simulink model "ModelConveyorWithLogic"  (R2020b)
settings: Solver=FixedStepAuto  StartTime=0.0  StopTime=Inf  FixedStep=0.010  RelTol=1e-3
libraries: simulink x2
settings Model: Creator=kaebi  LastModifiedBy=kaebi
settings OptimizationCC: DefaultParameterBehavior=Inlined  LocalBlockOutputs=off
settings RTWCC: Description=TwinCAT GRT Target  SystemTargetFile=TwinCatGrt.tlc  GenCodeOnly=on  TemplateMakefile=tcgrt_msbuild.tmf  TargetLang=C++
settings STFCustomTargetCC: TargetLangStandard=C++03 (ISO)  ConcurrentExecutionCompliant=off  CombineOutputUpdateFcns=on  CodeInterfacePackaging=Reusable function  GRTInterface=off  GenerateAllocFcn=on  SystemTargetFile=TwinCatGrt.tlc
settings GRTTargetCC: TargetLangStandard=C++03 (ISO)  ParMdlRefBuildCompliant=off  CompOptLevelCompliant=off  ConcurrentExecutionCompliant=off  MatFileLogging=off  CodeInterfacePackaging=Reusable function  GenerateAllocFcn=on  UseToolchainInfoCompliant=off  ExtModeMexFile=TcExtModeClient

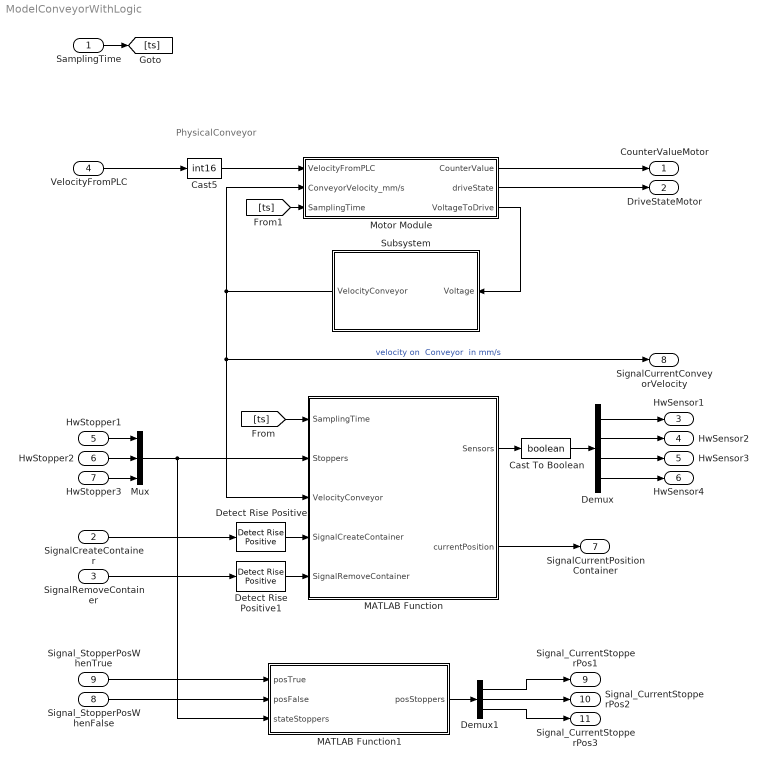
== system ModelConveyorWithLogic ==
  note: PhysicalConveyor
  SamplingTime : Inport
  SignalCreateContainer : Inport  Port=2  OutDataTypeStr=boolean
  SignalRemoveContainer : Inport  Port=3  OutDataTypeStr=boolean
  VelocityFromPLC : Inport  Port=4  OutDataTypeStr=int16
  HwStopper1 : Inport  Port=5  OutDataTypeStr=boolean
  HwStopper2 : Inport  Port=6  OutDataTypeStr=boolean
  HwStopper3 : Inport  Port=7  OutDataTypeStr=boolean
  Signal_StopperPosWhenFalse : Inport  Port=8
  Signal_StopperPosWhenTrue : Inport  Port=9
  Cast To Boolean : DataTypeConversion  OutDataTypeStr=boolean
  Cast5 : DataTypeConversion  OutDataTypeStr=int16
  Demux : Demux
  Demux1 : Demux  Outputs=3
  Detect Rise Positive : simulink/Logic and Bit Operations/Detect Rise Positive  vinit=0  OutDataTypeStr=boolean
  Detect Rise Positive1 : simulink/Logic and Bit Operations/Detect Rise Positive  vinit=0  OutDataTypeStr=boolean
  MATLAB Function : MATLAB Function  TreatAsAtomicUnit=on
  MATLAB Function1 : MATLAB Function  TreatAsAtomicUnit=on
  Motor Module : Subsystem
  Mux : Mux  Inputs=3
  Subsystem : Subsystem
  CounterValueMotor : Outport
  DriveStateMotor : Outport  Port=2
  HwSensor1 : Outport  Port=3
  HwSensor2 : Outport  Port=4
  HwSensor3 : Outport  Port=5
  HwSensor4 : Outport  Port=6
  SignalCurrentPositionContainer : Outport  Port=7
  SignalCurrentConveyorVelocity : Outport  Port=8
  Signal_CurrentStopperPos1 : Outport  Port=9
  Signal_CurrentStopperPos2 : Outport  Port=10
  Signal_CurrentStopperPos3 : Outport  Port=11
  wires:
  Subsystem/1(VelocityConveyor) -> SignalCurrentConveyorVelocity/1, MATLAB Function/3(VelocityConveyor), Motor Module/2(ConveyorVelocity_mm/s)  "velocity on  Conveyor  in mm/s"
  Detect Rise Positive1/1 -> MATLAB Function/5(SignalRemoveContainer)
  SignalRemoveContainer/1 -> Detect Rise Positive1/1
  HwStopper3/1 -> Mux/3
  Mux/1 -> MATLAB Function1/3(stateStoppers), MATLAB Function/2(Stoppers)
  HwStopper1/1 -> Mux/1
  MATLAB Function/2(currentPosition) -> SignalCurrentPositionContainer/1
  Detect Rise Positive/1 -> MATLAB Function/4(SignalCreateContainer)
  Motor Module/3(VoltageToDrive) -> Subsystem/1(Voltage)
  [ts] -> MATLAB Function/1(SamplingTime)
  Cast5/1 -> Motor Module/1(VelocityFromPLC)
  Motor Module/2(driveState) -> DriveStateMotor/1
  [ts] -> Motor Module/3(SamplingTime)
  VelocityFromPLC/1 -> Cast5/1
  SignalCreateContainer/1 -> Detect Rise Positive/1
  HwStopper2/1 -> Mux/2
  Motor Module/1(CounterValue) -> CounterValueMotor/1
  SamplingTime/1 -> [ts]
  Demux/4 -> HwSensor4/1
  Demux/3 -> HwSensor3/1
  Demux/2 -> HwSensor2/1
  Demux/1 -> HwSensor1/1
  MATLAB Function/1(Sensors) -> Cast To Boolean/1
  MATLAB Function1/1(posStoppers) -> Demux1/1
  Demux1/1 -> Signal_CurrentStopperPos1/1
  Demux1/2 -> Signal_CurrentStopperPos2/1
  Demux1/3 -> Signal_CurrentStopperPos3/1
  Signal_StopperPosWhenTrue/1 -> MATLAB Function1/1(posTrue)
  Signal_StopperPosWhenFalse/1 -> MATLAB Function1/2(posFalse)
  Cast To Boolean/1 -> Demux/1

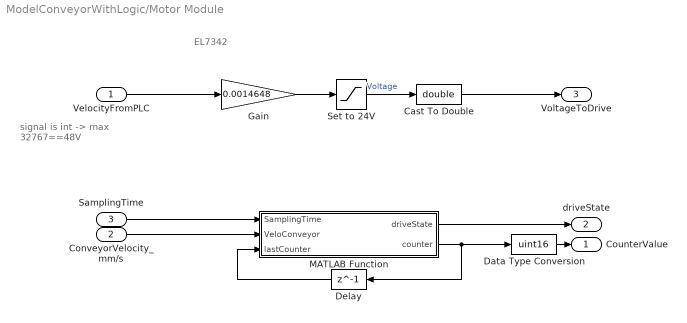
== system ModelConveyorWithLogic/Motor Module ==
  note: signal is int ->
      | max 32767==48V
  note: EL7342
  VelocityFromPLC : Inport
  ConveyorVelocity_mm/s : Inport  Port=2
  SamplingTime : Inport  Port=3
  Cast To Double : DataTypeConversion  OutDataTypeStr=double
  Data Type Conversion : DataTypeConversion  OutDataTypeStr=uint16
  Delay : Delay  DelayLength=1
  Gain : Gain  Gain=0.0014648
  MATLAB Function : MATLAB Function  TreatAsAtomicUnit=on
  Set to 24V : Saturate  UpperLimit=24  LowerLimit=-24
  CounterValue : Outport
  driveState : Outport  Port=2
  VoltageToDrive : Outport  Port=3
  wires:
  Gain/1 -> Set to 24V/1
  Cast To Double/1 -> VoltageToDrive/1
  ConveyorVelocity_mm/s/1 -> MATLAB Function/2(VeloConveyor)
  MATLAB Function/1(driveState) -> driveState/1
  Set to 24V/1 -> Cast To Double/1  "Voltage"
  Delay/1 -> MATLAB Function/3(lastCounter)
  SamplingTime/1 -> MATLAB Function/1(SamplingTime)
  VelocityFromPLC/1 -> Gain/1
  Data Type Conversion/1 -> CounterValue/1
  MATLAB Function/2(counter) -> Delay/1, Data Type Conversion/1

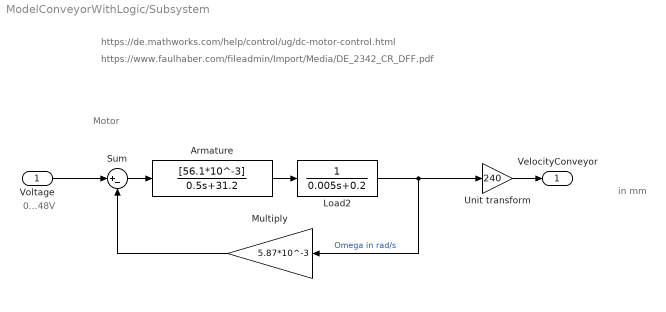
== system ModelConveyorWithLogic/Subsystem ==
  note: Motor
  note: in mm
  note: https://de.mathworks.com/help/control/ug/dc-motor-control.html
  note: 0...48V
  note: https://www.faulhaber.com/fileadmin/Import/Media/DE_2342_CR_DFF.pdf
  Voltage : Inport
  Armature : TransferFcn  Numerator=[56.1*10^-3]  Denominator=[0.5 31.2]
  Load2 : TransferFcn  Denominator=[0.005 0.2]
  Multiply : Gain  Gain=5.87*10^-3
  Sum : Sum  Inputs=|+-
  Unit transform : Gain  Gain=240
  VelocityConveyor : Outport
  wires:
  Unit transform/1 -> VelocityConveyor/1
  Armature/1 -> Load2/1
  Voltage/1 -> Sum/1
  Sum/1 -> Armature/1
  Load2/1 -> Unit transform/1, Multiply/1  "Omega in rad/s"
  Multiply/1 -> Sum/2

== matlab function ModelConveyorWithLogic/MATLAB Function ==
  settings: updateMethod=DISCRETE
  data: SamplingTime input; Stoppers input; Sensors output size=[1 4]; VelocityConveyor input; SignalCreateContainer input; SignalRemoveContainer input; currentPosition output
function [Sensors, currentPosition]  = Logic(SamplingTime, Stoppers, VelocityConveyor, SignalCreateContainer, SignalRemoveContainer)
%% Interface
% Stoppers = [ stopper1, stopper2, stopper3];
% Sensors = [Sensor1, Sensor2, Sensor3, Sensor4
% VelocityConveyor ... current velocity in mm/s

%% Variables
persistent containerPos;
if (isempty(containerPos))
    containerPos = -1;
end

StoppingPos1 = 120;
StoppingPos2 = 240;
StoppingPos3 = 360;
EndPosition = 600;

SensorPos1 = 09;
SensorPos2 = 19;
SensorPos3 = 29;
SensorPos4 = 39;
SensorRangePlusMinus = 1.5;

Sensors = zeros(1,4);
currentPosition = -2;

%% Create and Remove
if (SignalCreateContainer && containerPos == -1)
    containerPos = 0;
end

if (SignalRemoveContainer && containerPos == EndPosition)
    containerPos = -1;
end


%% Logic Movement
newPos = containerPos + VelocityConveyor*SamplingTime;

if (containerPos < 0 )    
elseif (containerPos <= StoppingPos1)
    if (newPos > StoppingPos1 && Stoppers(1) == false)
        containerPos = StoppingPos1;
    else
        containerPos = newPos;
    end  
elseif (containerPos <= StoppingPos2)
    if (newPos > StoppingPos2 && Stoppers(2) == false)
        containerPos = StoppingPos2;
    else
        containerPos = newPos;
    end    
elseif (containerPos <= StoppingPos3)
    if (newPos > StoppingPos3 && Stoppers(3) == false)
        containerPos = StoppingPos3;
    else
        containerPos = newPos;
    end  
    
elseif (containerPos <= EndPosition)
    if (newPos > EndPosition)
        containerPos = EndPosition;
    else
        containerPos = newPos;
    end  
end

% output Value
currentPosition = containerPos;

%% Logic Sensors
if (containerPos > SensorPos1-SensorRangePlusMinus && containerPos < SensorPos1+SensorRangePlusMinus) 
    Sensors(1) = 1;
elseif (containerPos > SensorPos2-SensorRangePlusMinus && containerPos < SensorPos2+SensorRangePlusMinus)
    Sensors(2) = 1;
elseif (containerPos > SensorPos3-SensorRangePlusMinus && containerPos < SensorPos3+SensorRangePlusMinus)
    Sensors(3) = 1;
elseif (containerPos > SensorPos4-SensorRangePlusMinus && containerPos < SensorPos4+SensorRangePlusMinus)
    Sensors(4) = 1;
end

== matlab function ModelConveyorWithLogic/Motor Module/MATLAB Function ==
  data: driveState output; SamplingTime input; VeloConveyor input; counter output; lastCounter input
function [driveState,counter] = fcn(SamplingTime, VeloConveyor, lastCounter)
%%
%    VeloConveyor in mm/s
%    SamplingTime in s
%    lastCounter 1count = 0.0001mm

%%
driveState = uint8(0);
driveState = bitset(driveState,1,1);    % Ready to enable
driveState = bitset(driveState,2,1);    % Ready 
if (VeloConveyor > 0)
    driveState = bitset(driveState,5,1);    % Moving Positive
elseif (VeloConveyor < 0)
    driveState = bitset(driveState,6,1);    % Moving Negative
end

diff = VeloConveyor*SamplingTime*10000;
if (lastCounter+diff >= 65535)
    counter = lastCounter+diff -65535;
else
    counter = lastCounter + VeloConveyor*SamplingTime*10000;
end

end

== matlab function ModelConveyorWithLogic/MATLAB Function1 ==
  data: posTrue input; posStoppers output; posFalse input; stateStoppers input
function posStoppers  = CalcStopperPos(posTrue, posFalse, stateStoppers)

posStoppers = stateStoppers;
posStoppers(stateStoppers==1) = posTrue;
posStoppers(stateStoppers==0) = posFalse;
